simulink model "bh_lag_quad_TEST_LINEAR_SYS_CONT_DESIGN"  (R2017a)
settings: Solver=ode23t  StartTime=0.0  StopTime=77  RelTol=1e-5
values from neighbouring files (symbols this model uses):
  K = [1.17115605021e-19 -1.34457008772e-16 -7.12795123873e-18 0.0431836511993 -1.6541551896e-12 -1.73191982917e-16 0.126584124772 -3.94383892487e-18 1.65419671556e-12 0.126584124772 -1.82762947107e-16 -8.51651764895e-17 ... (60 elements, 4x15)]    [OLD_bh_CONT_DES_RESULTS_LQI_quadcopter.mat]    (also in bh_CONT_DES_RESULTS_LQI_quadcopter.mat = [2.6635655919e-18 -4.41749299763e-16 -1.11640474601e-16 0.04)
undefined symbols (not defined in the file or in its folder): A, B, C, D, P_veh, sigbuilder_block, x0
libraries: simulink_extras x2, simulink x2
settings Model: Creator=bhorton  LastModifiedBy=bhorton
settings SolverCC: ZeroCrossAlgorithm=Adaptive

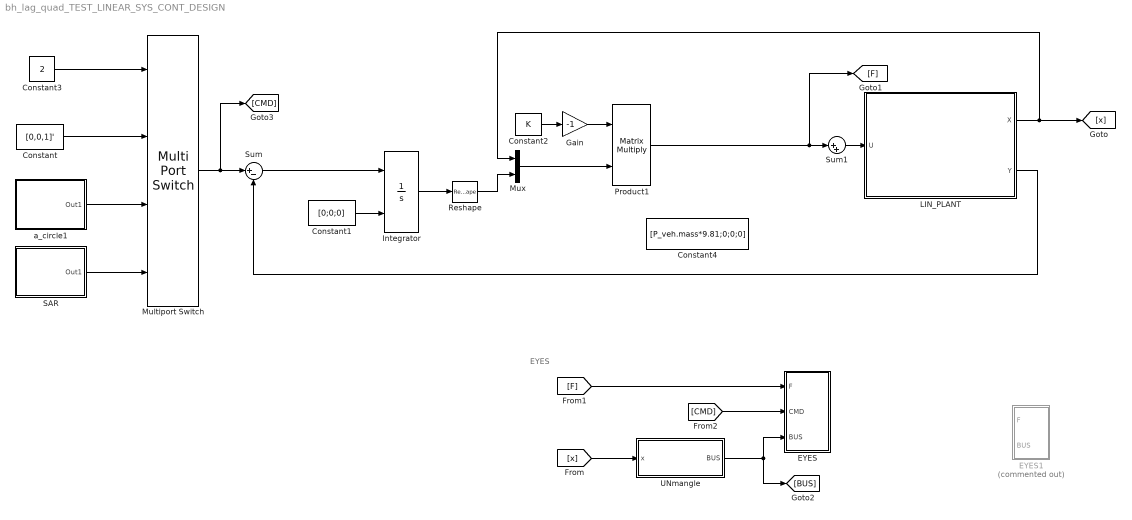
== system bh_lag_quad_TEST_LINEAR_SYS_CONT_DESIGN ==
  note: EYES
  Constant : Constant  Value=[0,0,1]'  VectorParams1D=off
  Constant1 : Constant  Value=[0;0;0]  VectorParams1D=off
  Constant2 : Constant  Value=K  VectorParams1D=off
  Constant3 : Constant  Value=2
  Constant4 : Constant  Value=[P_veh.mass*9.81;0;0;0]
  EYES : Subsystem
  EYES1 : Subsystem  Commented=on
  Gain : Gain  Gain=-1
  Integrator : Integrator  InitialConditionSource=external
  LIN_PLANT : Subsystem
  Multiport Switch : MultiPortSwitch
  Mux : Mux  Inputs=2
  Product1 : Product  Multiplication=Matrix(*)
  Reshape : Reshape  OutputDimensionality=Column vector (2-D)
  SAR : Subsystem
  Sum : Sum  Inputs=|+-
  Sum1 : Sum  Inputs=|++
  UNmangle : Subsystem
  a_circle1 : Subsystem
  wires:
  Sum/1 -> Integrator/1
  Constant1/1 -> Integrator/2
  Integrator/1 -> Reshape/1
  LIN_PLANT/1(X) -> [x], Mux/1
  Reshape/1 -> Mux/2
  Constant2/1 -> Gain/1
  Gain/1 -> Product1/1
  Mux/1 -> Product1/2
  LIN_PLANT/2(Y) -> Sum/2
  [x] -> UNmangle/1(x)
  Sum1/1 -> LIN_PLANT/1(U)
  Product1/1 -> Sum1/1, [F]
  UNmangle/1(BUS) -> [BUS], EYES/3(BUS)
  [F] -> EYES/1(F)
  Multiport Switch/1 -> [CMD], Sum/1
  a_circle1/1(Out1) -> Multiport Switch/3
  SAR/1(Out1) -> Multiport Switch/4
  Constant/1 -> Multiport Switch/2
  Constant3/1 -> Multiport Switch/1
  [CMD] -> EYES/2("CMD ")

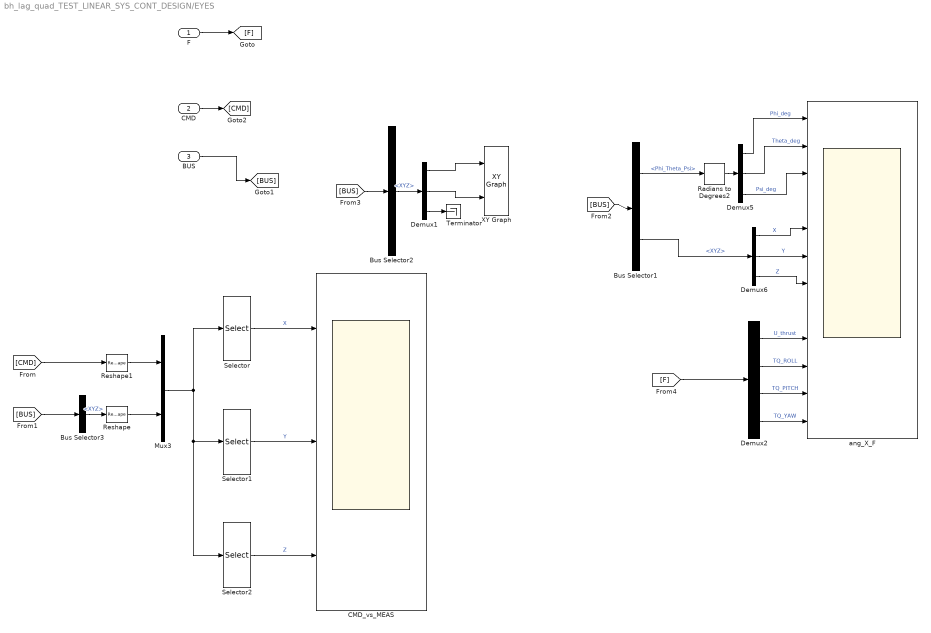
== system bh_lag_quad_TEST_LINEAR_SYS_CONT_DESIGN/EYES ==
  F : Inport
  "CMD " : Inport  Port=2
  BUS : Inport  Port=3
  Bus Selector1 : BusSelector  OutputSignals=Phi_Theta_Psi,XYZ
  Bus Selector2 : BusSelector  OutputSignals=XYZ
  Bus Selector3 : BusSelector  OutputSignals=XYZ
  CMD_vs_MEAS : Scope  NumInputPorts=3
  Demux1 : Demux  Outputs=3
  Demux2 : Demux
  Demux5 : Demux  Outputs=3
  Demux6 : Demux  Outputs=3
  Mux3 : Mux  Inputs=2
  Radians to Degrees2 : simulink_extras/Transformations/Radians to Degrees
  Reshape : Reshape  OutputDimensionality=Column vector (2-D)
  Reshape1 : Reshape  OutputDimensionality=Column vector (2-D)
  Selector : Selector  InputPortWidth=6  IndexOptions=Index vector (dialog)  Indices=[1 4]  OutputSizes=1
  Selector1 : Selector  InputPortWidth=6  IndexOptions=Index vector (dialog)  Indices=[2 5]  OutputSizes=1
  Selector2 : Selector  InputPortWidth=6  IndexOptions=Index vector (dialog)  Indices=[3 6]  OutputSizes=1
  Terminator : Terminator
  XY Graph : simulink/Sinks/XY Graph  xmin=-3  xmax=3  ymin=-3  ymax=3  st=-1
  ang_X_F : Scope  NumInputPorts=12
  wires:
  BUS/1 -> [BUS]
  F/1 -> [F]
  Demux1/3 -> Terminator/1
  Bus Selector2/1 -> Demux1/1  "<XYZ>"
  Demux1/1 -> XY Graph/1
  Bus Selector1/2 -> Demux6/1  "<XYZ>"
  [BUS] -> Bus Selector1/1
  Demux5/2 -> ang_X_F/2  "Theta_deg"
  [F] -> Demux2/1
  Demux6/2 -> ang_X_F/6  "Y"
  Demux5/3 -> ang_X_F/3  "Psi_deg"
  Demux1/2 -> XY Graph/2
  Radians to Degrees2/1 -> Demux5/1
  Demux5/1 -> ang_X_F/1  "Phi_deg"
  [BUS] -> Bus Selector2/1
  Demux6/1 -> ang_X_F/5  "X"
  Demux6/3 -> ang_X_F/7  "Z"
  Bus Selector1/1 -> Radians to Degrees2/1  "<Phi_Theta_Psi>"
  Demux2/1 -> ang_X_F/9  "U_thrust"
  Demux2/2 -> ang_X_F/10  "TQ_ROLL"
  Demux2/3 -> ang_X_F/11  "TQ_PITCH"
  Demux2/4 -> ang_X_F/12  "TQ_YAW"
  "CMD "/1 -> [CMD]
  Selector2/1 -> CMD_vs_MEAS/3  "Z"
  Selector1/1 -> CMD_vs_MEAS/2  "Y"
  Selector/1 -> CMD_vs_MEAS/1  "X"
  [BUS] -> Bus Selector3/1
  Bus Selector3/1 -> Reshape/1  "<XYZ>"
  [CMD] -> Reshape1/1
  Reshape1/1 -> Mux3/1
  Reshape/1 -> Mux3/2
  Mux3/1 -> Selector1/1, Selector2/1, Selector/1

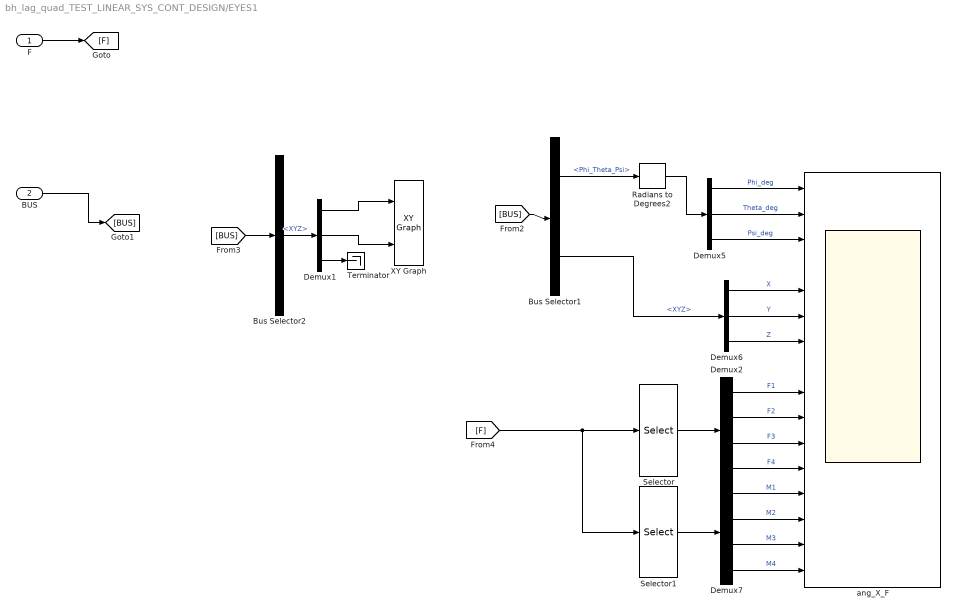
== system bh_lag_quad_TEST_LINEAR_SYS_CONT_DESIGN/EYES1 ==
  F : Inport
  BUS : Inport  Port=2
  Bus Selector1 : BusSelector  OutputSignals=Phi_Theta_Psi,XYZ
  Bus Selector2 : BusSelector  OutputSignals=XYZ
  Demux1 : Demux  Outputs=3
  Demux2 : Demux
  Demux5 : Demux  Outputs=3
  Demux6 : Demux  Outputs=3
  Demux7 : Demux
  Radians to Degrees2 : simulink_extras/Transformations/Radians to Degrees
  Selector : Selector  InputPortWidth=8  IndexOptions=Index vector (dialog)  Indices=1:4  OutputSizes=1
  Selector1 : Selector  InputPortWidth=8  IndexOptions=Index vector (dialog)  Indices=5:8  OutputSizes=1
  Terminator : Terminator
  XY Graph : simulink/Sinks/XY Graph  xmin=-3  xmax=3  ymin=-3  ymax=3  st=-1
  ang_X_F : Scope  NumInputPorts=16
  wires:
  BUS/1 -> [BUS]
  F/1 -> [F]
  Demux2/4 -> ang_X_F/12  "F4"
  Demux1/3 -> Terminator/1
  Bus Selector2/1 -> Demux1/1  "<XYZ>"
  Selector1/1 -> Demux7/1
  Demux1/1 -> XY Graph/1
  Bus Selector1/2 -> Demux6/1  "<XYZ>"
  Demux7/3 -> ang_X_F/15  "M3"
  [F] -> Selector1/1, Selector/1
  [BUS] -> Bus Selector1/1
  Demux5/2 -> ang_X_F/2  "Theta_deg"
  Selector/1 -> Demux2/1
  Demux6/2 -> ang_X_F/6  "Y"
  Demux5/3 -> ang_X_F/3  "Psi_deg"
  Demux1/2 -> XY Graph/2
  Radians to Degrees2/1 -> Demux5/1
  Demux5/1 -> ang_X_F/1  "Phi_deg"
  Demux7/2 -> ang_X_F/14  "M2"
  Demux2/1 -> ang_X_F/9  "F1"
  Demux2/2 -> ang_X_F/10  "F2"
  [BUS] -> Bus Selector2/1
  Demux2/3 -> ang_X_F/11  "F3"
  Demux7/1 -> ang_X_F/13  "M1"
  Demux7/4 -> ang_X_F/16  "M4"
  Demux6/1 -> ang_X_F/5  "X"
  Demux6/3 -> ang_X_F/7  "Z"
  Bus Selector1/1 -> Radians to Degrees2/1  "<Phi_Theta_Psi>"

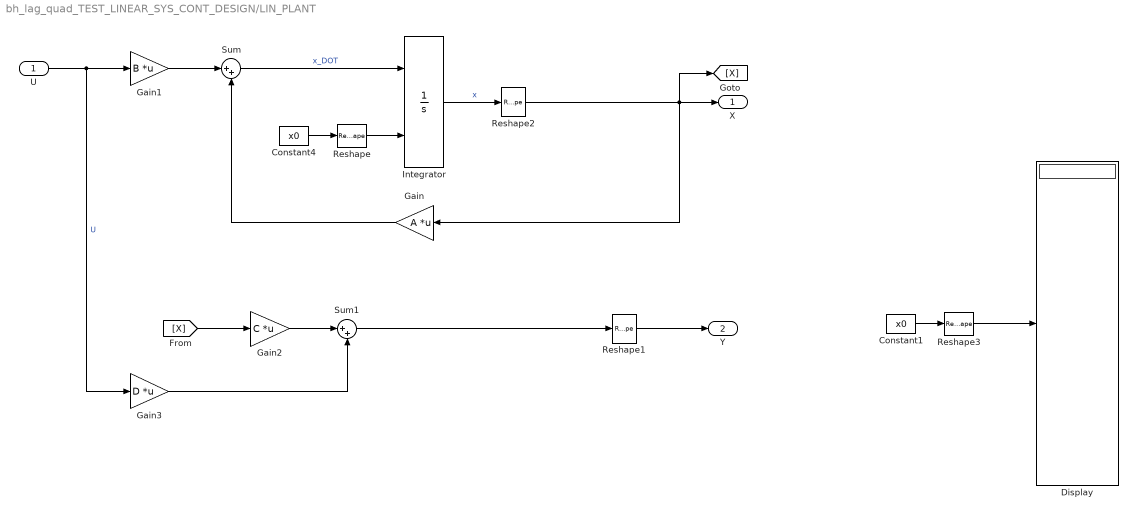
== system bh_lag_quad_TEST_LINEAR_SYS_CONT_DESIGN/LIN_PLANT ==
  U : Inport
  Constant1 : Constant  Value=x0
  Constant4 : Constant  Value=x0
  Display : Display
  Gain : Gain  Gain=A  Multiplication=Matrix(K*u)
  Gain1 : Gain  Gain=B  Multiplication=Matrix(K*u)
  Gain2 : Gain  Gain=C  Multiplication=Matrix(K*u)
  Gain3 : Gain  Gain=D  Multiplication=Matrix(K*u)
  Integrator : Integrator  InitialConditionSource=external
  Reshape{,1..3} (4 alike) : Reshape  OutputDimensionality=Column vector (2-D)
  Sum : Sum  Inputs=|++
  Sum1 : Sum  Inputs=|++
  X : Outport
  Y : Outport  Port=2
  wires:
  Reshape/1 -> Integrator/2
  Constant4/1 -> Reshape/1
  Sum/1 -> Integrator/1  "x_DOT"
  U/1 -> Gain3/1, Gain1/1  "U"
  Gain1/1 -> Sum/1
  Integrator/1 -> Reshape2/1  "x"
  Sum1/1 -> Reshape1/1
  Reshape2/1 -> [X], X/1, Gain/1
  Reshape1/1 -> Y/1
  Constant1/1 -> Reshape3/1
  Reshape3/1 -> Display/1
  Gain/1 -> Sum/2
  [X] -> Gain2/1
  Gain2/1 -> Sum1/1
  Gain3/1 -> Sum1/2

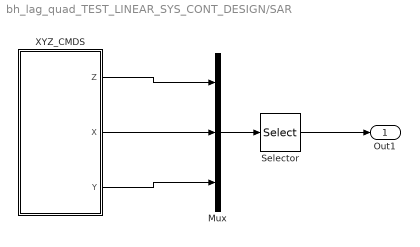
== system bh_lag_quad_TEST_LINEAR_SYS_CONT_DESIGN/SAR ==
  Mux : Mux  Inputs=3
  Selector : Selector  InputPortWidth=3  IndexOptions=Index vector (dialog)  Indices=[2 3 1]  OutputSizes=1
  XYZ_CMDS : Subsystem  Tag=STV Subsys  LoadFcn=sigbuilder_block('load');  StartFcn=sigbuilder_block('start');  StopFcn=sigbuilder_block('stop');  ClipboardFcn=sigbuilder_block('clipboard');  mask(Sigbuilder block){tuvar=[0:10]}
      mask help: Simulink:masks:SigbuilderBlock_MD
      mask init:
      | if ~strcmp(get_param(bdroot(gcbh),'SimulationStatus'),'stopped') tuvar = sigbuilder_block('maskInit'); end
      settings: CopyFcn=sigbuilder_block('copy');  DeleteFcn=sigbuilder_block('delete');  ModelCloseFcn=sigbuilder_block('modelClose');  PreSaveFcn=sigbuilder_block('preSave');  PauseFcn=sigbuilder_block('pause');  ContinueFcn=sigbuilder_block('continue');  NameChangeFcn=sigbuilder_block('namechange');  OpenFcn=sigbuilder_block('open',[189 32.25 551.25 400.5 ]);  CloseFcn=sigbuilder_block('close');
      mask Display: plot(0, 0, 100, 100,[2, 2, 32, 32, 2], [68, 8, 8, 68, 68],[32, 2], [38, 38], [32, 19, 2],[53, 60, 44], [32, 17, 17, 2],[16, 16, 31, 31]);txt = getActiveGroup(gcbh);text(2, 100, txt,'verticalAlignment', 'top');
  Out1 : Outport
  wires:
  XYZ_CMDS/3(Y) -> Mux/3
  XYZ_CMDS/1(Z) -> Mux/1
  XYZ_CMDS/2(X) -> Mux/2
  Mux/1 -> Selector/1
  Selector/1 -> Out1/1

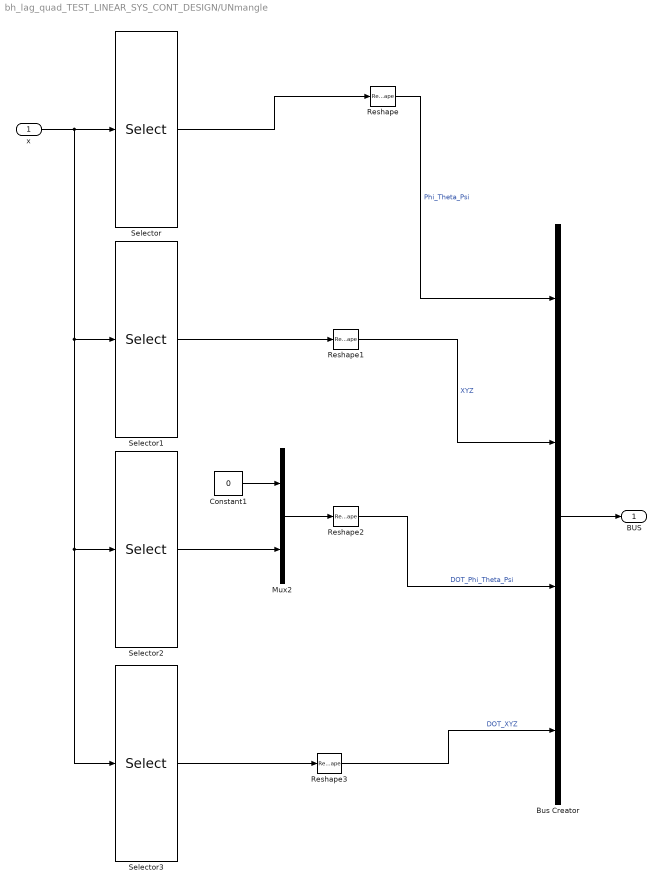
== system bh_lag_quad_TEST_LINEAR_SYS_CONT_DESIGN/UNmangle ==
  x : Inport
  Bus Creator : BusCreator  Inputs=4
  Constant1 : Constant  Value=0  VectorParams1D=off
  Mux2 : Mux  Inputs=2
  Reshape{,1..3} (4 alike) : Reshape  OutputDimensionality=Column vector (2-D)
  Selector : Selector  InputPortWidth=12  IndexOptions=Index vector (dialog)  Indices=7:9  OutputSizes=1
  Selector1 : Selector  InputPortWidth=12  IndexOptions=Index vector (dialog)  Indices=10:12  OutputSizes=1
  Selector2 : Selector  InputPortWidth=12  IndexOptions=Index vector (dialog)  Indices=1:3  OutputSizes=1
  Selector3 : Selector  InputPortWidth=12  IndexOptions=Index vector (dialog)  Indices=4:6  OutputSizes=1
  BUS : Outport
  wires:
  x/1 -> Selector3/1, Selector2/1, Selector1/1, Selector/1
  Selector/1 -> Reshape/1
  Selector1/1 -> Reshape1/1
  Selector2/1 -> Mux2/2
  Constant1/1 -> Mux2/1
  Mux2/1 -> Reshape2/1
  Selector3/1 -> Reshape3/1
  Bus Creator/1 -> BUS/1
  Reshape/1 -> Bus Creator/1  "Phi_Theta_Psi"
  Reshape1/1 -> Bus Creator/2  "XYZ"
  Reshape2/1 -> Bus Creator/3  "DOT_Phi_Theta_Psi"
  Reshape3/1 -> Bus Creator/4  "DOT_XYZ"

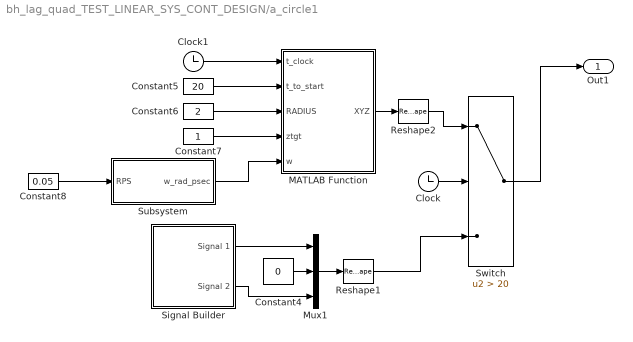
== system bh_lag_quad_TEST_LINEAR_SYS_CONT_DESIGN/a_circle1 ==
  Clock : Clock
  Clock1 : Clock
  Constant4 : Constant  Value=0  VectorParams1D=off
  Constant5 : Constant  Value=20  VectorParams1D=off
  Constant6 : Constant  Value=2  VectorParams1D=off
  Constant7 : Constant  VectorParams1D=off
  Constant8 : Constant  Value=0.05  VectorParams1D=off
  MATLAB Function : MATLAB Function  TreatAsAtomicUnit=on
  Mux1 : Mux  Inputs=3
  Reshape1 : Reshape  OutputDimensionality=Column vector (2-D)
  Reshape2 : Reshape  OutputDimensionality=Column vector (2-D)
  Signal Builder : Subsystem  Tag=STV Subsys  LoadFcn=sigbuilder_block('load');  StartFcn=sigbuilder_block('start');  StopFcn=sigbuilder_block('stop');  ClipboardFcn=sigbuilder_block('clipboard');  mask(Sigbuilder block){tuvar=[0:10]}
      mask help: Simulink:masks:SigbuilderBlock_MD
      mask init:
      | if ~strcmp(get_param(bdroot(gcbh),'SimulationStatus'),'stopped') tuvar = sigbuilder_block('maskInit'); end
      settings: CopyFcn=sigbuilder_block('copy');  DeleteFcn=sigbuilder_block('delete');  ModelCloseFcn=sigbuilder_block('modelClose');  PreSaveFcn=sigbuilder_block('preSave');  PauseFcn=sigbuilder_block('pause');  ContinueFcn=sigbuilder_block('continue');  NameChangeFcn=sigbuilder_block('namechange');  OpenFcn=sigbuilder_block('open',[437.6 199.2 550.4 400 ]);  CloseFcn=sigbuilder_block('close');
      mask Display: plot(0, 0, 100, 100,[2, 2, 32, 32, 2], [68, 8, 8, 68, 68],[32, 2], [38, 38], [32, 19, 2],[53, 60, 44], [32, 17, 17, 2],[16, 16, 31, 31]);txt = getActiveGroup(gcbh);text(2, 100, txt,'verticalAlignment', 'top');
  Subsystem : Subsystem
  Switch : Switch  Criteria=u2 > Threshold  Threshold=20
  Out1 : Outport
  wires:
  Switch/1 -> Out1/1
  MATLAB Function/1(XYZ) -> Reshape2/1
  Constant6/1 -> MATLAB Function/3(RADIUS)
  Constant7/1 -> MATLAB Function/4(ztgt)
  Subsystem/1(w_rad_psec) -> MATLAB Function/5(w)
  Constant5/1 -> MATLAB Function/2(t_to_start)
  Reshape1/1 -> Switch/3
  Constant4/1 -> Mux1/2
  Signal Builder/1(Signal 1) -> Mux1/1
  Signal Builder/2(Signal 2) -> Mux1/3
  Mux1/1 -> Reshape1/1
  Clock/1 -> Switch/2
  Clock1/1 -> MATLAB Function/1(t_clock)
  Constant8/1 -> Subsystem/1(RPS)
  Reshape2/1 -> Switch/1

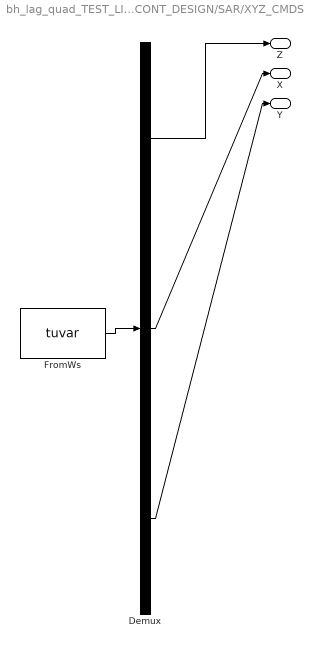
== system bh_lag_quad_TEST_LINEAR_SYS_CONT_DESIGN/SAR/XYZ_CMDS ==
  Demux : Demux  Tag=STV Demux  Outputs=3
  FromWs : FromWorkspace  Tag=STV FromWs  VariableName=tuvar  SampleTime=0
      SigBuilderData=|
      | common.afterFinalStr = 'Extrapolate'
      | common.sampleTime = 0
      | dataSet(1).timeRange = [0 200]
      | dataSet(1).name = 'small_steps'
      | dataSet(2).timeRange = [0 200]
      | dataSet(2).name = 'zStairs_xyConstVEL'
      | dataSet(3).timeRange = [0 500]
      | dataSet(3).name = 'sineWaves'
      | dataSet(4).timeRange = [0 200]
      | dataSet(4).name = 'ZERO'
      | dataSet(5).timeRange = [0 200]
      | dataSet(5).name = 'SEARCH_P1'
      | sbobj.Name = 'Signal Builder'
      | sbobj.Groups(1).Name = 'small_steps'
      | sbobj.Groups(1).Signals(1).Name = 'Z'
      | sbobj.Groups(1).Signals(1).XData = [0 10 10.000001 20 20.000001 30 30.000001 55 200]
      | sbobj.Groups(1).Signals(1).YData = [0 0 2 2 2 2 2 2 2]
      | sbobj.Groups(1).Signals(2).Name = 'X'
      | sbobj.Groups(1).Signals(2).XData = [0 10 10.000001 20 20.000001 30 30.000001 55 200]
      | sbobj.Groups(1).Signals(2).YData = [0 0 0 0 3 3 3 3 3]
      | sbobj.Groups(1).Signals(3).Name = 'Y'
      | sbobj.Groups(1).Signals(3).XData = [0 10 10.000001 20 20.000001 30 30.000001 55 200]
      | sbobj.Groups(1).Signals(3).YData = [0 0 0 0 0 0 1 1 1]
      | sbobj.Groups(1).TimeRange = [0 200]
      | sbobj.Groups(2).Name = 'zStairs_xyConstVEL'
      | sbobj.Groups(2).Signals(1).Name = 'Z'
      | sbobj.Groups(2).Signals(1).XData = [0 10 10.000001 20 20.000001 30 30.000001 40 40.000001 55 200]
      | sbobj.Groups(2).Signals(1).YData = [0 0 1 1 2 2 1 1 0 0 0]
      | sbobj.Groups(2).Signals(2).Name = 'X'
      | sbobj.Groups(2).Signals(2).XData = [0 10 10.000001 20 20.000001 30 30.000001 40 40.000001 55 200]
      | sbobj.Groups(2).Signals(2).YData = [0 1 1.0000001 2 2.0000001 3 3.0000001 4 4.0000001 5.5 20]
      | sbobj.Groups(2).Signals(3).Name = 'Y'
      | sbobj.Groups(2).Signals(3).XData = [0 10 10.000001 20 20.000001 30 30.000001 40 40.000001 55 200]
      | sbobj.Groups(2).Signals(3).YData = [0 0.5 0.50000005 1 1.00000005 1.5 1.50000005 2 2.00000005 2.75 10]
      | sbobj.Groups(2).TimeRange = [0 200]
      | sbobj.Groups(3).Name = 'sineWaves'
      | sbobj.Groups(3).Signals(1).Name = 'Z'
      | sbobj.Groups(3).Signals(1).XData = [0 0.1 0.2 0.3 0.4 0.5 0.6 0.7 0.8 0.9 1 1.1 ... (5001 elements, 1x5001)]
      | sbobj.Groups(3).Signals(1).YData = [0 0.0314107325553 0.0627904665622 0.0941082340641 0.125333128258 0.156434333994 0.18738115819 0.218143060119 0.248689681547 0.278990876699 0.309016742004 0.338737645607 ... (5001 elements, 1x5001)]
      | sbobj.Groups(3).Signals(2).Name = 'X'
      | sbobj.Groups(3).Signals(2).XData = [0 0.1 0.2 0.3 0.4 0.5 0.6 0.7 0.8 0.9 1 1.1 ... (5001 elements, 1x5001)]
      | sbobj.Groups(3).Signals(2).YData = [0 0.01 0.02 0.03 0.04 0.05 0.06 0.07 0.08 0.09 0.1 0.11 ... (5001 elements, 1x5001)]
      | sbobj.Groups(3).Signals(3).Name = 'Y'
      | sbobj.Groups(3).Signals(3).XData = [0 0.1 0.2 0.3 0.4 0.5 0.6 0.7 0.8 0.9 1 1.1 ... (5001 elements, 1x5001)]
      | sbobj.Groups(3).Signals(3).YData = [0 0.0157073040455 0.0314107325553 0.04710641095 0.0627904665622 0.0784590295926 0.0941082340641 0.109734218776 0.125333128258 0.140901113717 0.156434333994 0.171928956505 ... (5001 elements, 1x5001)]
      | sbobj.Groups(3).TimeRange = [0 500]
      | sbobj.Groups(4).Name = 'ZERO'
      | sbobj.Groups(4).Signals(1).Name = 'Z'
      | sbobj.Groups(4).Signals(1).XData = [0 200]
      | sbobj.Groups(4).Signals(1).YData = [0 0]
      | sbobj.Groups(4).Signals(2).Name = 'X'
      | sbobj.Groups(4).Signals(2).XData = [0 200]
      | sbobj.Groups(4).Signals(2).YData = [0 0]
      | sbobj.Groups(4).Signals(3).Name = 'Y'
      | sbobj.Groups(4).Signals(3).XData = [0 200]
      | sbobj.Groups(4).Signals(3).YData = [0 0]
      | sbobj.Groups(4).TimeRange = [0 200]
      | sbobj.Groups(5).Name = 'SEARCH_P1'
      | sbobj.Groups(5).Signals(1).Name = 'Z'
      | sbobj.Groups(5).Signals(1).XData = [0 7 27 32 52 57 77 82 102 107 127 132 157 187 200]
      | sbobj.Groups(5).Signals(1).YData = [0 5 5 5 5 5 5 5 5 5 5 5 5 0 0]
      | sbobj.Groups(5).Signals(2).Name = 'X'
      | sbobj.Groups(5).Signals(2).XData = [0 7 27 32 52 57 77 82 102 107 127 132 157 187 200]
      | sbobj.Groups(5).Signals(2).YData = [0 5 25 25 5 5 25 25 5 5 25 25 0 0 0]
      | sbobj.Groups(5).Signals(3).Name = 'Y'
      | sbobj.Groups(5).Signals(3).XData = [0 7 27 32 52 57 77 82 102 107 127 132 157 187 200]
      | sbobj.Groups(5).Signals(3).YData = [0 5 5 10 10 15 15 20 20 25 25 30 30 0 0]
      | sbobj.Groups(5).TimeRange = [0 200]
  Z : Outport
  X : Outport  Tag=STV Outport  Port=2
  Y : Outport  Tag=STV Outport  Port=3
  wires:
  Demux/1 -> Z/1
  FromWs/1 -> Demux/1
  Demux/2 -> X/1
  Demux/3 -> Y/1

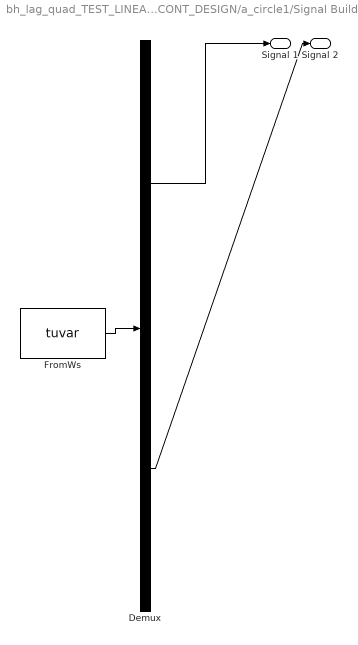
== system bh_lag_quad_TEST_LINEAR_SYS_CONT_DESIGN/a_circle1/Signal Builder ==
  Demux : Demux  Tag=STV Demux  Outputs=2
  FromWs : FromWorkspace  Tag=STV FromWs  VariableName=tuvar  SampleTime=0
      SigBuilderData=|
      | common.afterFinalStr = 'Extrapolate'
      | common.sampleTime = 0
      | dataSet.timeRange = [0 22]
      | dataSet.name = 'Group 1'
      | sbobj.Groups.Name = 'Group 1'
      | sbobj.Groups.Signals(1).Name = 'Signal 1'
      | sbobj.Groups.Signals(1).XData = [0 7.95 7.95 22]
      | sbobj.Groups.Signals(1).YData = [0 0 1.99 1.98]
      | sbobj.Groups.Signals(2).Name = 'Signal 2'
      | sbobj.Groups.Signals(2).XData = [0 12 16 22]
      | sbobj.Groups.Signals(2).YData = [0 0 1 1]
      | sbobj.Groups.TimeRange = [0 22]
  Signal 1 : Outport  Tag=STV Outport
  Signal 2 : Outport  Tag=STV Outport  Port=2
  wires:
  Demux/1 -> Signal 1/1
  FromWs/1 -> Demux/1
  Demux/2 -> Signal 2/1

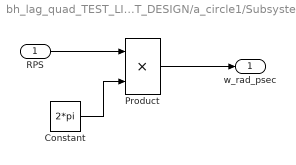
== system bh_lag_quad_TEST_LINEAR_SYS_CONT_DESIGN/a_circle1/Subsystem ==
  RPS : Inport
  Constant : Constant  Value=2*pi
  Product : Product  Inputs=**
  w_rad_psec : Outport
  wires:
  Constant/1 -> Product/2
  RPS/1 -> Product/1
  Product/1 -> w_rad_psec/1

== matlab function bh_lag_quad_TEST_LINEAR_SYS_CONT_DESIGN/a_circle1/MATLAB Function ==
  data: t_clock input; XYZ output; t_to_start input; RADIUS input; ztgt input; w input
function XYZ = fcn(t_clock, t_to_start, RADIUS, ztgt, w)

t    = t_clock - t_to_start;

theta = w*t;

x = RADIUS * cos(theta);
y = RADIUS * sin(theta);
z = ztgt;


XYZ = [x;y;z];
